simulink model "c_lab4sim"  (R2020b)
settings: Solver=FixedStepAuto  StartTime=0.0  StopTime=50  FixedStep=0.001  RelTol=1e-3
settings Model: Creator=musa oğural  LastModifiedBy=musa oğural

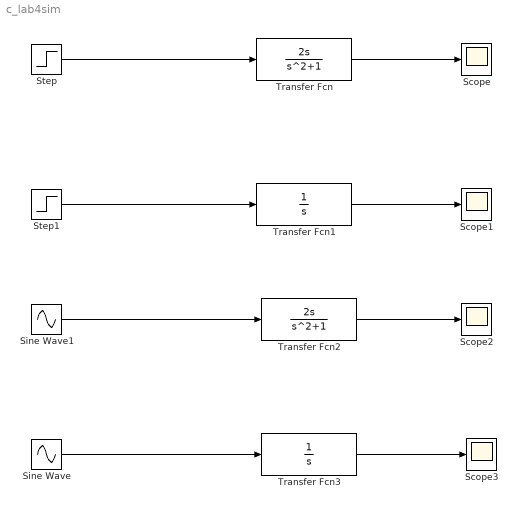
== system c_lab4sim ==
  Scope{,1..3} (4 alike) : Scope
  Sine Wave : Sin  SampleTime=0
  Sine Wave1 : Sin  SampleTime=0
  Step : Step  Time=0  SampleTime=0
  Step1 : Step  Time=0  SampleTime=0
  Transfer Fcn : TransferFcn  Numerator=[2 0]  Denominator=[1 0 1]
  Transfer Fcn1 : TransferFcn  Denominator=[1 0 ]
  Transfer Fcn2 : TransferFcn  Numerator=[2 0]  Denominator=[1 0 1]
  Transfer Fcn3 : TransferFcn  Denominator=[1 0 ]
  wires:
  Step1/1 -> Transfer Fcn1/1
  Transfer Fcn1/1 -> Scope1/1
  Step/1 -> Transfer Fcn/1
  Transfer Fcn/1 -> Scope/1
  Sine Wave1/1 -> Transfer Fcn2/1
  Transfer Fcn2/1 -> Scope2/1
  Sine Wave/1 -> Transfer Fcn3/1
  Transfer Fcn3/1 -> Scope3/1
